simulink model "pid_test"  (R2022b)
settings: Solver=VariableStepAuto  StartTime=0.0  StopTime=10  RelTol=1e-3
undefined symbols (not defined in the file): c_s, k_s, k_t, kd, ki, kp, m_s, m_u
settings Model: Creator=user  LastModifiedBy=user

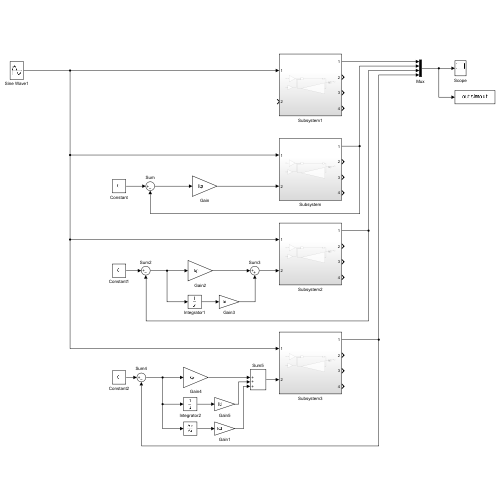
[thumbnail: Simulink's stored preview of the top-level diagram]
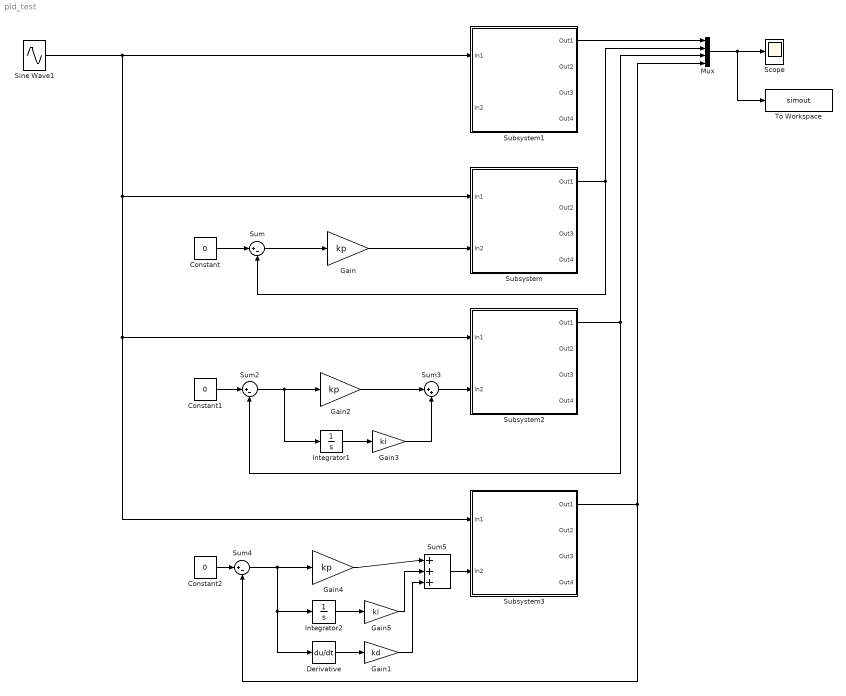
== system pid_test ==
  Constant : Constant  Value=0
  Constant1 : Constant  Value=0
  Constant2 : Constant  Value=0
  Derivative : Derivative
  Gain : Gain  Gain=kp
  Gain1 : Gain  Gain=kd
  Gain2 : Gain  Gain=kp
  Gain3 : Gain  Gain=ki
  Gain4 : Gain  Gain=kp
  Gain5 : Gain  Gain=ki
  Integrator1 : Integrator
  Integrator2 : Integrator
  Mux : Mux
  Scope : Scope
  Sine Wave1 : Sin  Amplitude=0.03  Frequency=4*pi  SampleTime=0
  Subsystem : Subsystem
  Subsystem1 : Subsystem
  Subsystem2 : Subsystem
  Subsystem3 : Subsystem
  Sum : Sum  Inputs=|+-
  Sum2 : Sum  Inputs=|+-
  Sum3 : Sum  Inputs=|++
  Sum4 : Sum  Inputs=|+-
  Sum5 : Sum  Inputs=|+++
  To Workspace : ToWorkspace  VariableName=simout  SampleTime=-1
  wires:
  Sine Wave1/1 -> Subsystem1/1(In1), Subsystem/1(In1), Subsystem3/1(In1), Subsystem2/1(In1)
  Subsystem/1(Out1) -> Sum/2, Mux/2
  Constant/1 -> Sum/1
  Sum/1 -> Gain/1
  Subsystem1/1(Out1) -> Mux/1
  Mux/1 -> Scope/1, To Workspace/1
  Gain3/1 -> Sum3/2
  Sum3/1 -> Subsystem2/2(In2)
  Integrator1/1 -> Gain3/1
  Gain2/1 -> Sum3/1
  Sum2/1 -> Gain2/1, Integrator1/1
  Constant1/1 -> Sum2/1
  Constant2/1 -> Sum4/1
  Sum4/1 -> Derivative/1, Integrator2/1, Gain4/1
  Gain4/1 -> Sum5/1
  Integrator2/1 -> Gain5/1
  Sum5/1 -> Subsystem3/2(In2)
  Gain5/1 -> Sum5/2
  Gain/1 -> Subsystem/2(In2)
  Subsystem2/1(Out1) -> Mux/3, Sum2/2
  Subsystem3/1(Out1) -> Mux/4, Sum4/2
  Derivative/1 -> Gain1/1
  Gain1/1 -> Sum5/3

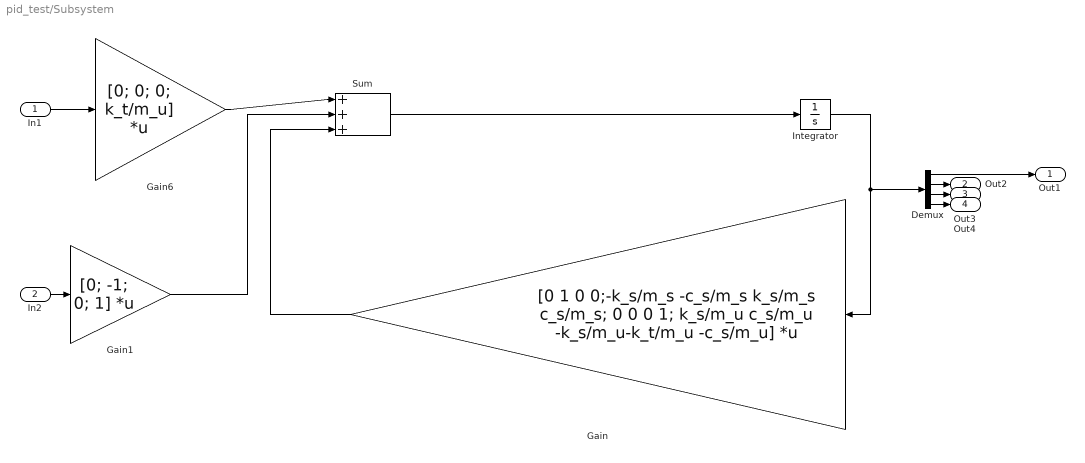
== system pid_test/Subsystem ==
  In1 : Inport
  In2 : Inport  Port=2
  Demux : Demux
  Gain : Gain  Gain=[0 1 0 0;-k_s/m_s -c_s/m_s k_s/m_s c_s/m_s; 0 0 0 1; k_s/m_u c_s/m_u -k_s/m_u-k_t/m_u -c_s/m_u]  Multiplication=Matrix(K*u)
  Gain1 : Gain  Gain=[0; -1; 0; 1]  Multiplication=Matrix(K*u)
  Gain6 : Gain  Gain=[0; 0; 0; k_t/m_u]  Multiplication=Matrix(K*u)
  Integrator : Integrator
  Sum : Sum  Inputs=|+++
  Out1 : Outport
  Out2 : Outport  Port=2
  Out3 : Outport  Port=3
  Out4 : Outport  Port=4
  wires:
  In2/1 -> Gain1/1
  Gain1/1 -> Sum/2
  Gain6/1 -> Sum/1
  Integrator/1 -> Demux/1, Gain/1
  Demux/2 -> Out2/1
  Gain/1 -> Sum/3
  Sum/1 -> Integrator/1
  Demux/4 -> Out4/1
  Demux/1 -> Out1/1
  In1/1 -> Gain6/1
  Demux/3 -> Out3/1

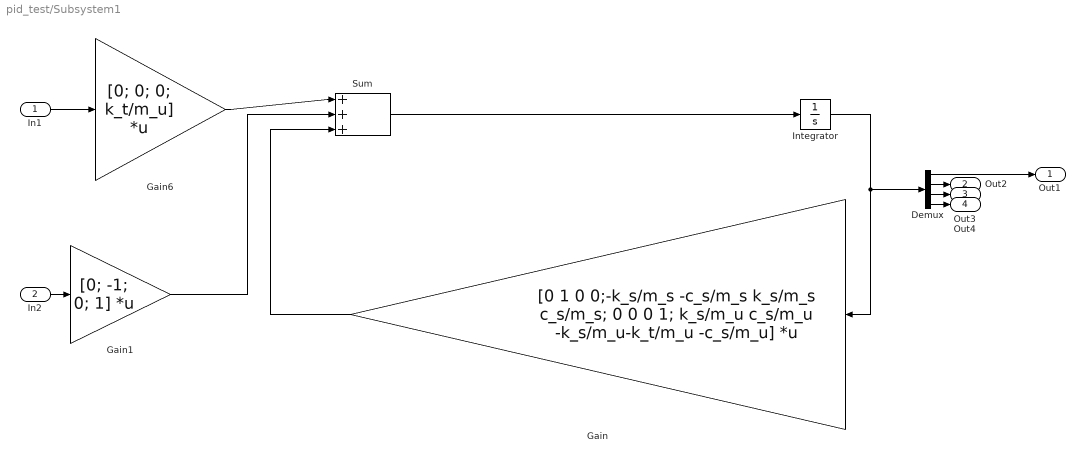
== system pid_test/Subsystem1 ==
  In1 : Inport
  In2 : Inport  Port=2
  Demux : Demux
  Gain : Gain  Gain=[0 1 0 0;-k_s/m_s -c_s/m_s k_s/m_s c_s/m_s; 0 0 0 1; k_s/m_u c_s/m_u -k_s/m_u-k_t/m_u -c_s/m_u]  Multiplication=Matrix(K*u)
  Gain1 : Gain  Gain=[0; -1; 0; 1]  Multiplication=Matrix(K*u)
  Gain6 : Gain  Gain=[0; 0; 0; k_t/m_u]  Multiplication=Matrix(K*u)
  Integrator : Integrator
  Sum : Sum  Inputs=|+++
  Out1 : Outport
  Out2 : Outport  Port=2
  Out3 : Outport  Port=3
  Out4 : Outport  Port=4
  wires:
  Demux/3 -> Out3/1
  In1/1 -> Gain6/1
  Demux/1 -> Out1/1
  Demux/4 -> Out4/1
  Sum/1 -> Integrator/1
  Gain/1 -> Sum/3
  Demux/2 -> Out2/1
  Integrator/1 -> Gain/1, Demux/1
  Gain6/1 -> Sum/1
  Gain1/1 -> Sum/2
  In2/1 -> Gain1/1

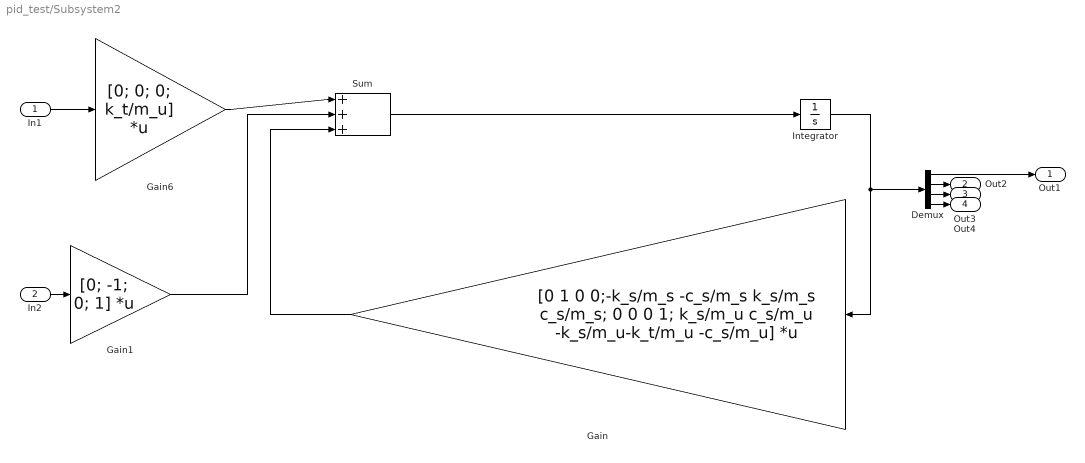
== system pid_test/Subsystem2 ==
  In1 : Inport
  In2 : Inport  Port=2
  Demux : Demux
  Gain : Gain  Gain=[0 1 0 0;-k_s/m_s -c_s/m_s k_s/m_s c_s/m_s; 0 0 0 1; k_s/m_u c_s/m_u -k_s/m_u-k_t/m_u -c_s/m_u]  Multiplication=Matrix(K*u)
  Gain1 : Gain  Gain=[0; -1; 0; 1]  Multiplication=Matrix(K*u)
  Gain6 : Gain  Gain=[0; 0; 0; k_t/m_u]  Multiplication=Matrix(K*u)
  Integrator : Integrator
  Sum : Sum  Inputs=|+++
  Out1 : Outport
  Out2 : Outport  Port=2
  Out3 : Outport  Port=3
  Out4 : Outport  Port=4
  wires:
  Demux/3 -> Out3/1
  In1/1 -> Gain6/1
  Demux/1 -> Out1/1
  Demux/4 -> Out4/1
  Sum/1 -> Integrator/1
  Gain/1 -> Sum/3
  Demux/2 -> Out2/1
  Integrator/1 -> Gain/1, Demux/1
  Gain6/1 -> Sum/1
  Gain1/1 -> Sum/2
  In2/1 -> Gain1/1

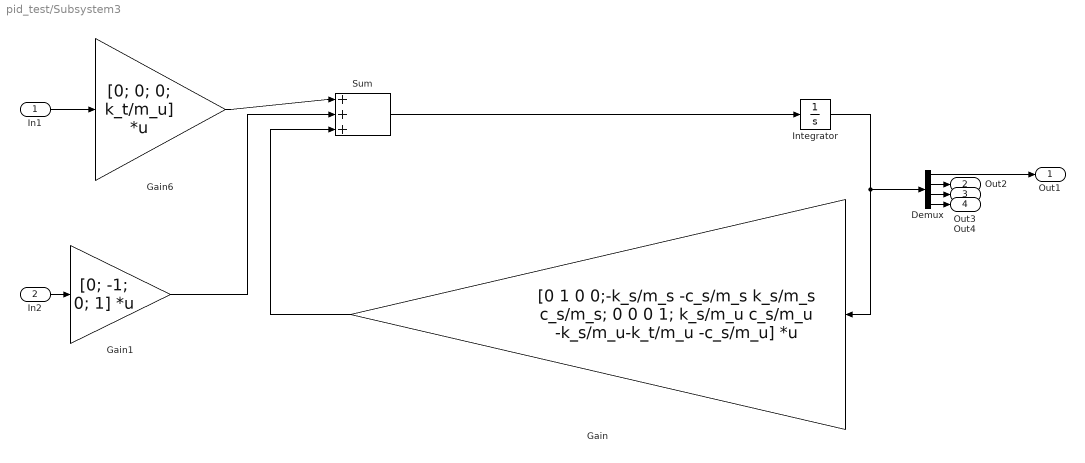
== system pid_test/Subsystem3 ==
  In1 : Inport
  In2 : Inport  Port=2
  Demux : Demux
  Gain : Gain  Gain=[0 1 0 0;-k_s/m_s -c_s/m_s k_s/m_s c_s/m_s; 0 0 0 1; k_s/m_u c_s/m_u -k_s/m_u-k_t/m_u -c_s/m_u]  Multiplication=Matrix(K*u)
  Gain1 : Gain  Gain=[0; -1; 0; 1]  Multiplication=Matrix(K*u)
  Gain6 : Gain  Gain=[0; 0; 0; k_t/m_u]  Multiplication=Matrix(K*u)
  Integrator : Integrator
  Sum : Sum  Inputs=|+++
  Out1 : Outport
  Out2 : Outport  Port=2
  Out3 : Outport  Port=3
  Out4 : Outport  Port=4
  wires:
  In2/1 -> Gain1/1
  Gain1/1 -> Sum/2
  Gain6/1 -> Sum/1
  Integrator/1 -> Demux/1, Gain/1
  Demux/2 -> Out2/1
  Gain/1 -> Sum/3
  Sum/1 -> Integrator/1
  Demux/4 -> Out4/1
  Demux/1 -> Out1/1
  In1/1 -> Gain6/1
  Demux/3 -> Out3/1
